simulink model "lab1_symulacja"  (R2022a)
settings: Solver=VariableStepAuto  StartTime=0.0  StopTime=10  RelTol=1e-3
settings Model: Creator=rober  LastModifiedBy=rober

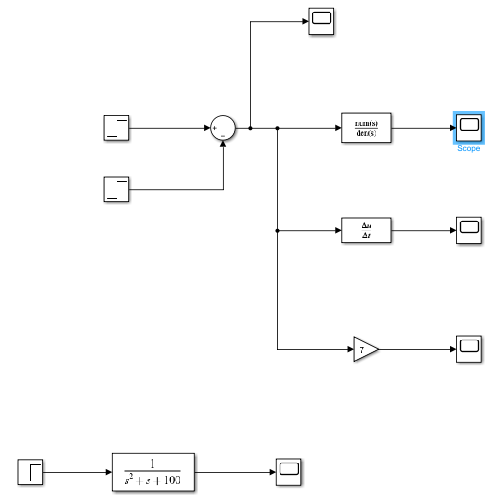
[thumbnail: Simulink's stored preview of the top-level diagram]
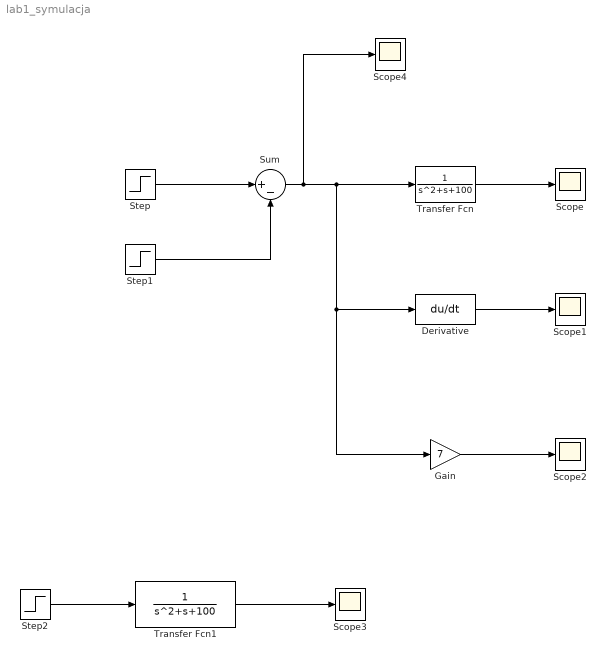
== system lab1_symulacja ==
  Derivative : Derivative
  Gain : Gain  Gain=7
  Scope{,1..4} (5 alike) : Scope
  Step : Step  After=1/0.0001  SampleTime=0
  Step1 : Step  Time=1.0001  After=1/0.0001  SampleTime=0
  Step2 : Step  SampleTime=0
  Sum : Sum  Inputs=|+-
  Transfer Fcn : TransferFcn  Denominator=[1 1 100]
  Transfer Fcn1 : TransferFcn  Denominator=[1 1 100]
  wires:
  Step/1 -> Sum/1
  Step1/1 -> Sum/2
  Sum/1 -> Scope4/1, Gain/1, Derivative/1, Transfer Fcn/1
  Transfer Fcn/1 -> Scope/1
  Derivative/1 -> Scope1/1
  Gain/1 -> Scope2/1
  Transfer Fcn1/1 -> Scope3/1
  Step2/1 -> Transfer Fcn1/1
